simulink model "PID"  (R2023a)
settings: Solver=VariableStepAuto  StartTime=0  StopTime=5  RelTol=1e-3
model workspace (MAT data in the model file):
  mu = [0 0.4 0.8 0.97 1 0.98 0.96 0.94 0.92 0.9 0.88 0.855 0.83 0.81 0.79 0.77 0.75 0.73 0.72 0.71 0.7]
  slip = [0 0.05 0.1 0.15 0.2 0.25 0.3 0.35 0.4 0.45 0.5 0.55 0.6 0.65 0.7 0.75 0.8 0.85 0.9 0.95 1]
libraries: slpidlib x1, spsCurrentMeasurementLib x1, spsDCVoltageSourceLib x1, spsPermanentMagnetSynchronousMachineLib x1, spsUniversalBridgeLib x1, simulink x1, spspowerguiLib x1
settings Model: Creator=13524  LastModifiedBy=13524

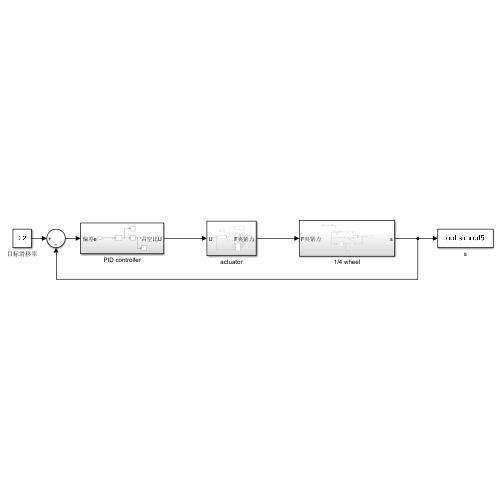
[thumbnail: Simulink's stored preview of the top-level diagram]
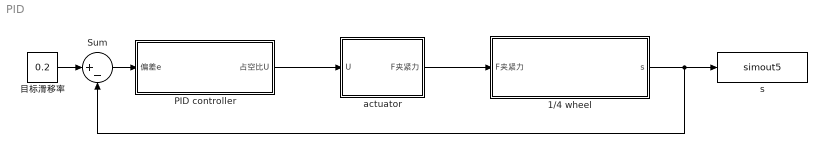
== system PID ==
  1/4 wheel : Subsystem
  PID controller : Subsystem
  Sum : Sum  Inputs=|+-
  actuator : Subsystem
  s : ToWorkspace  VariableName=simout5  SaveFormat=Timeseries  SampleTime=-1
  目标滑移率 : Constant  Value=0.2
  wires:
  1/4 wheel/1(s) -> s/1, Sum/2
  目标滑移率/1 -> Sum/1
  Sum/1 -> PID controller/1(偏差e)
  PID controller/1(占空比U) -> actuator/1(U)
  actuator/1(F夹紧力) -> 1/4 wheel/1(F夹紧力)

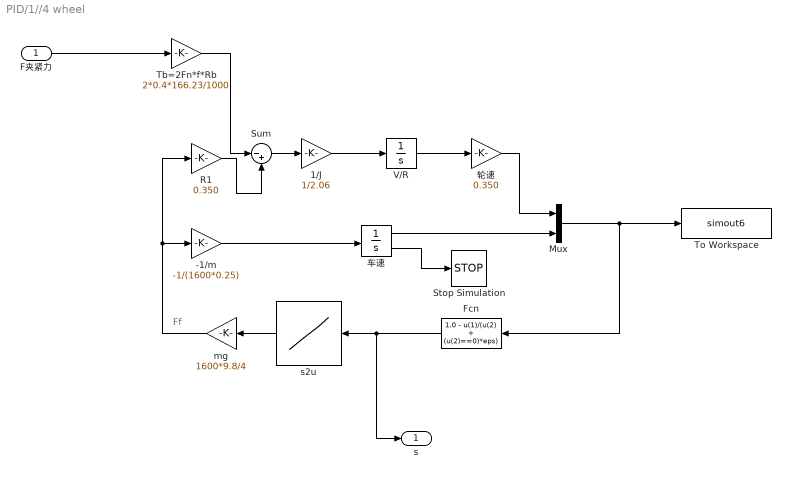
== system PID/1//4 wheel ==
  note: Ff
  F夹紧力 : Inport
  -1/m : Gain  Gain=-1/(1600*0.25)
  1/J : Gain  Gain=1/2.06
  Fcn : Fcn  Expr=1.0 - u(1)/(u(2) + (u(2)==0)*eps)
  Mux : Mux  Inputs=2
  R1 : Gain  Gain=0.350
  Stop Simulation : Stop
  Sum : Sum  Inputs=|-+
  Tb=2Fn*f*Rb : Gain  Gain=2*0.4*166.23/1000
  To Workspace : ToWorkspace  VariableName=simout6  SaveFormat=Timeseries  SampleTime=-1
  V/R : Integrator  InitialCondition=40/0.350  LimitOutput=on  UpperSaturationLimit=1000  LowerSaturationLimit=0
  mg : Gain  Gain=1600*9.8/4
  s2u : Lookup_n-D  NumberOfTableDimensions=1  BreakpointsForDimension1=[0;0.05;0.1;0.15;0.2;0.25;0.3;0.35;0.4;0.45;0.5;0.55;0.6;0.65;0.7;0.75;0.8;0.85;0.9;0.95;1]  Table=[0;0.4;0.8;0.97;1;0.98;0.96;0.94;0.92;0.9;0.88;0.855;0.83;0.81;0.79;0.77;0.75;0.73;0.72;0.71;0.7]  InternalRulePriority=Speed  RndMeth=Simplest
  车速 : Integrator  InitialCondition=40  LimitOutput=on  UpperSaturationLimit=100  LowerSaturationLimit=0  ShowSaturationPort=on
  轮速 : Gain  Gain=0.350
  s : Outport
  wires:
  V/R/1 -> 轮速/1
  轮速/1 -> Mux/1
  车速/1 -> Mux/2
  Mux/1 -> To Workspace/1, Fcn/1
  Fcn/1 -> s/1, s2u/1
  s2u/1 -> mg/1
  -1/m/1 -> 车速/1
  mg/1 -> R1/1, -1/m/1
  R1/1 -> Sum/2
  Sum/1 -> 1/J/1
  车速/2 -> Stop Simulation/1
  1/J/1 -> V/R/1
  F夹紧力/1 -> Tb=2Fn*f*Rb/1
  Tb=2Fn*f*Rb/1 -> Sum/1

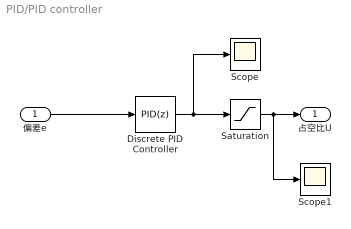
== system PID/PID controller ==
  偏差e : Inport
  Discrete PID Controller : slpidlib/PID Controller  Controller=PID  Form=Parallel  TimeDomain=Discrete-time  UseExternalTs=off  SampleTime=-1  IntegratorMethod=Forward Euler  FilterMethod=Forward Euler  ControllerParametersSource=internal  P=100  I=150  UseKiTs=off  D=0.2  N=100  UseFilter=off  TunerSelectOption=Transfer Function Based (PID Tuner App)  InitialConditionSource=internal  InitialConditionForIntegrator=0  InitialConditionForFilter=0  DifferentiatorICPrevScaledInput=0  ExternalReset=none  TrackingMode=off  Kt=1  LimitOutput=off  SatLimitsSource=internal  UpperSaturationLimit=inf  LowerSaturationLimit=-inf  LinearizeAsGain=off  AntiWindupMode=none  Kb=1  LimitIntegrator=off  UpperIntegratorSaturationLimit=inf  LowerIntegratorSaturationLimit=-inf  POutMin=[]  POutMax=[]  IOutMin=[]  IOutMax=[]  DOutMin=[]  DOutMax=[]  NOutMin=[]  NOutMax=[]  SumOutMin=[]  SumOutMax=[]  SaturationOutMin=[]  SaturationOutMax=[]  PParamMin=[]  PParamMax=[]  IParamMin=[]  IParamMax=[]  DParamMin=[]  DParamMax=[]  NParamMin=[]  NParamMax=[]  KbParamMin=[]  KbParamMax=[]  KtParamMin=[]  KtParamMax=[]  KbOutMin=[]  KbOutMax=[]  KtOutMin=[]  KtOutMax=[]  IntegratorOutMin=[]  IntegratorOutMax=[]  FilterOutMin=[]  FilterOutMax=[]  SumI1OutMin=[]  SumI1OutMax=[]  SumI2OutMin=[]  SumI2OutMax=[]  SumI3OutMin=[]  SumI3OutMax=[]  SumI4OutMin=[]  SumI4OutMax=[]  SumDOutMin=[]  SumDOutMax=[]  DifferentiatorOutMin=[]  DifferentiatorOutMax=[]  FilterDiffOutCoefMin=[]  FilterDiffOutCoefMax=[]  ReciprocalOutMin=[]  ReciprocalOutMax=[]  SumDenOutMin=[]  SumDenOutMax=[]  SumNumOutMin=[]  SumNumOutMax=[]  DivideOutMin=[]  DivideOutMax=[]  UdiffTsProdOutMin=[]  UdiffTsProdOutMax=[]  NTsProdOutMin=[]  NTsProdOutMax=[]  UintegralTsProdOutMin=[]  UintegralTsProdOutMax=[]  UngainTsProdOutMin=[]  UngainTsProdOutMax=[]  ClampingZeroOutDataTypeStr=Inherit: Inherit via back propagation  ClampingZeroOutMin=[]  ClampingZeroOutMax=[]  FilterDenConstantOutDataTypeStr=Inherit: Inherit via back propagation  FilterDenConstantOutMin=[]  FilterDenConstantOutMax=[]  PCopyOutDataTypeStr=Inherit: Inherit via back propagation  PCopyOutMin=[]  PCopyOutMax=[]  NCopyOutDataTypeStr=Inherit: Inherit via back propagation  NCopyOutMin=[]  NCopyOutMax=[]  IntegratorContinuousStateAttributes=''  IntegratorStateMustResolveToSignalObject=off  IntegratorRTWStateStorageClass=Auto  FilterContinuousStateAttributes=''  FilterStateMustResolveToSignalObject=off  FilterRTWStateStorageClass=Auto  ParallelPVariant=InternalParameters  IdealPVariant=Disabled  IVariant=InternalParameters  DVariant=InternalParameters  IntegratorVariant=Discrete  SatVariant=Disabled  AWVariant=Passthrough  PCopyVariant=Disabled  TRVariant=Disabled  FdbkBlocksVariant=Forward  IdealPFdbkVariant=Disabled  SatFdbkVariant=Disabled  DerivativeFilterVariant=Differentiator  NVariant=Passthrough  NCopyVariant=Disabled_SignalSpec  FilterICVariant=InternalICsDifferentiator  IntegratorICVariant=InternalICs  ExternalResetVariant=Disabled  TRSumVariant=Passthrough  SumFdbkVariant=Disabled  SumVariant=Sum_PID  TsampFilterVariant=InternalTs  TsampNgainVariant=Passthrough  TsampIntegralVariant=Disabled_SignalSpec  ExternalSaturationOutDataTypeStr=Inherit: Same as second input
      settings: LibrarySourceBlock=simulink/Discrete/Discrete PID Controller
  Saturation : Saturate  UpperLimit=4  LowerLimit=-4
  Scope : Scope
  Scope1 : Scope
  占空比U : Outport
  wires:
  偏差e/1 -> Discrete PID Controller/1
  Discrete PID Controller/1 -> Scope/1, Saturation/1
  Saturation/1 -> Scope1/1, 占空比U/1

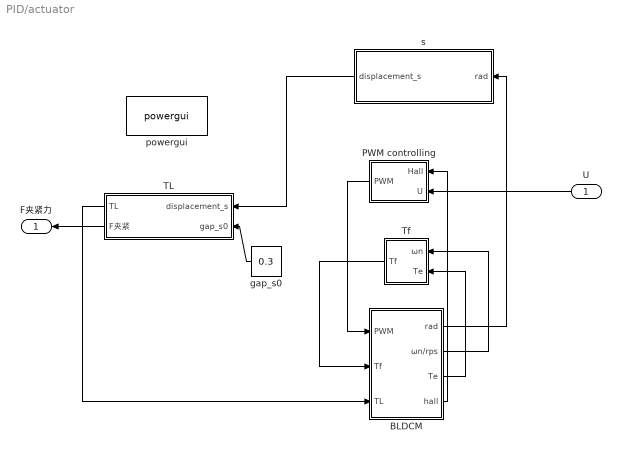
== system PID/actuator ==
  U : Inport
  BLDCM : Subsystem
  PWM controlling : Subsystem
  TL : Subsystem
  Tf : Subsystem
  gap_s0 : Constant  Value=0.3  VectorParams1D=off
  powergui : spspowerguiLib/powergui  Priority=1  SimulationMode=Discrete  SampleTime=0.0001  frequency=60  Iterations=50  frequencyindice=0  Pbase=100e6  ErrMax=1e-4  UnitsV=kV  UnitsW=MW  buscounter=0  FunctionMessages=off  echomessages=off  EnableUseOfTLC=off  CurrentSourceSwitches=off  DisableSnubberDevices=off  DisableRonSwitches=off  DisableVfSwitches=off  DisplayEquations=off  AutomaticDiscreteSolvers=off  SolverType=Tustin/Backward Euler (TBE)  Interpol=off  ExternalGateDelay=off  methode=off  Ts=100  x0status=blocks  SPID=on  SwTol=0  HookPort=off  NonlinearTolerance=1e-4  nMaxIteration=100  ContinueOnMaxIteration=off  RestoreLinks=warning  ResistiveCurrentMeasurement=off  Frange=[0:2:500]  Ylog=off  Xlog=on  ShowGrid=off  save=off  variable=ZData  structure=0  ZoomFFT=off  StartTime=0.0  cycles=1  DisplayStyle=1  fundamental=60  FreqAxis=off  MaxFrequency=1000  frequencyindicesteady=1  RmsSteady=1  display=off
  s : Subsystem
  F夹紧力 : Outport
  wires:
  PWM controlling/1(PWM) -> BLDCM/1(PWM)
  s/1(displacement_s) -> TL/1(displacement_s)
  BLDCM/4(hall) -> PWM controlling/1(Hall)
  Tf/1(Tf) -> BLDCM/2(Tf)
  TL/1(TL) -> BLDCM/3(TL)
  gap_s0/1 -> TL/2(gap_s0)
  BLDCM/1(rad) -> s/1(rad)
  BLDCM/3(Te) -> Tf/2(Te)
  BLDCM/2(ωn/rps) -> Tf/1(ωn)
  U/1 -> PWM controlling/2(U)
  TL/2(F夹紧) -> F夹紧力/1

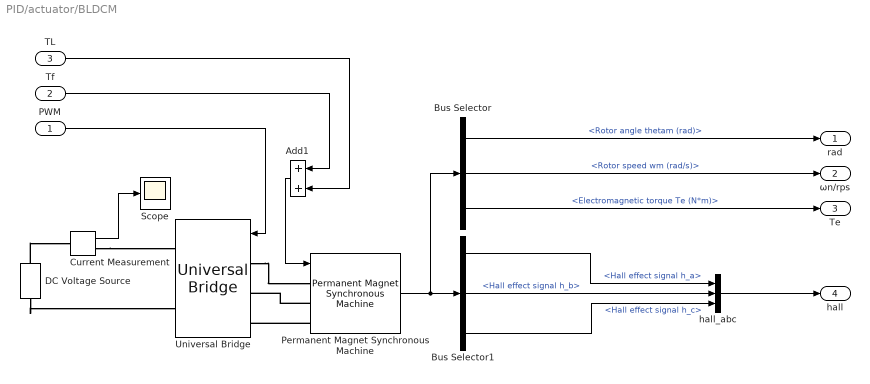
== system PID/actuator/BLDCM ==
  PWM : Inport
  Tf : Inport  Port=2
  TL : Inport  Port=3
  Add1 : Sum
  Bus Selector : BusSelector  OutputSignals=Rotor angle thetam (rad),Rotor speed wm (rad/s),Electromagnetic torque Te (N*m)
  Bus Selector1 : BusSelector  OutputSignals=Hall effect signal h_a,Hall effect signal h_b,Hall effect signal h_c
  Current Measurement : spsCurrentMeasurementLib/Current Measurement  PhasorSimulation=off  OutputType=Complex  PSBequivalent=0
  DC Voltage Source : spsDCVoltageSourceLib/DC Voltage Source  Amplitude=48  Measurements=Voltage
  Permanent Magnet Synchronous Machine : spsPermanentMagnetSynchronousMachineLib/Permanent Magnet Synchronous Machine  NbPhases=3  FluxDistribution=Trapezoidal  RotorType=Round  MechanicalLoad=Torque Tm  PresetModel=No  ShowDetailedParameters=on  MeasurementBus=off  Resistance=6.6  Inductance=0.99  dqInductances=[8.5e-3,8.5e-3]  La=0.000395  MachineConstant=Torque Constant (N.m / A_peak)  Flux=0.1405  VoltageCst=88.2788  TorqueCst=0.843  Flat=120  Mechanical=[0.00235 0.001086 3]  PolePairs=4  InitialConditions=[0,0,0,0]  InitialConditions5ph=[0 0 0 0 0 0]  RefAngle=Aligned with phase A axis (original Park)  IterativeDiscreteModel=Trapezoidal non iterative  TsBlock=-1  TsPowergui=0
  Scope : Scope
  Universal Bridge : spsUniversalBridgeLib/Universal Bridge  Arms=3  SnubberResistance=1e5  SnubberCapacitance=inf  Device=MOSFET / Diodes  Ron=1e-3  Lon=0  ForwardVoltages="[  0  0  ]"  ForwardVoltage=0  GTOparameters=[ 10e-6 , 20e-6 ]  IGBTparameters=[ 1e-6 , 2e-6 ]  Measurements=Device voltages  Measurements_2=None  converterType=Rectifier
  hall_abc : BusCreator  Inputs=3
  rad : Outport
  ωn/rps : Outport  Port=2
  Te : Outport  Port=3
  hall : Outport  Port=4
  wires:
  TL/1 -> Add1/2
  Bus Selector1/2 -> hall_abc/2  "<Hall effect signal h_b>"
  Add1/1 -> Permanent Magnet Synchronous Machine/1
  Bus Selector/3 -> Te/1  "<Electromagnetic torque Te (N*m)>"
  Bus Selector1/1 -> hall_abc/1  "<Hall effect signal h_a>"
  Permanent Magnet Synchronous Machine/1 -> Bus Selector/1, Bus Selector1/1
  Bus Selector1/3 -> hall_abc/3  "<Hall effect signal h_c>"
  Tf/1 -> Add1/1
  PWM/1 -> Universal Bridge/1
  Bus Selector/1 -> rad/1  "<Rotor angle thetam (rad)>"
  Bus Selector/2 -> ωn/rps/1  "<Rotor speed wm (rad/s)>"
  hall_abc/1 -> hall/1
  Current Measurement/1 -> Scope/1
  connections:
  Permanent Magnet Synchronous Machine/LConn3 -- Universal Bridge/LConn3
  Permanent Magnet Synchronous Machine/LConn2 -- Universal Bridge/LConn2
  Universal Bridge/LConn1 -- Permanent Magnet Synchronous Machine/LConn1
  DC Voltage Source/LConn1 -- Universal Bridge/RConn2
  DC Voltage Source/RConn1 -- Current Measurement/LConn1
  Current Measurement/RConn1 -- Universal Bridge/RConn1

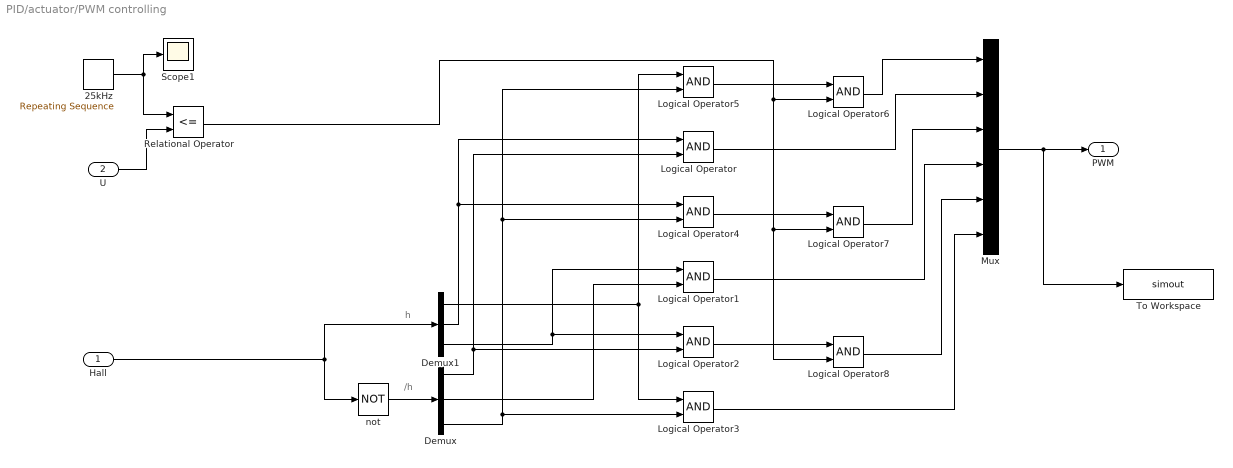
== system PID/actuator/PWM controlling ==
  note: h
  note: /h
  Hall : Inport
  U : Inport  Port=2
  25kHz : simulink/Sources/Repeating Sequence  rep_seq_t=[0 1/50000 1/25000]  rep_seq_y=[-4 4 -4]
  Demux : Demux  Outputs=3
  Demux1 : Demux  Outputs=3
  Logical Operator{,1..8} (9 alike) : Logic  AllPortsSameDT=off  OutDataTypeStr=boolean
  Mux : Mux  Inputs=6
  Relational Operator : RelationalOperator  Operator=<=  OutDataTypeStr=boolean  RndMeth=Simplest  InputSameDT=off
  Scope1 : Scope
  To Workspace : ToWorkspace  VariableName=simout  SaveFormat=Structure With Time  SampleTime=-1
  not : Logic  Operator=NOT  IconShape=distinctive  AllPortsSameDT=off  OutDataTypeStr=boolean
  PWM : Outport
  wires:
  Hall/1 -> not/1, Demux1/1
  Demux1/2 -> Logical Operator/1, Logical Operator4/1
  Demux/3 -> Logical Operator5/2, Logical Operator4/2, Logical Operator3/2
  Demux/1 -> Logical Operator/2, Logical Operator2/2
  Demux/2 -> Logical Operator1/2
  Logical Operator3/1 -> Mux/6
  Logical Operator7/1 -> Mux/3
  Relational Operator/1 -> Logical Operator6/2, Logical Operator7/2, Logical Operator8/2
  Demux1/1 -> Logical Operator5/1, Logical Operator3/1
  Demux1/3 -> Logical Operator1/1, Logical Operator2/1
  Logical Operator5/1 -> Logical Operator6/1
  Logical Operator8/1 -> Mux/5
  Logical Operator6/1 -> Mux/1
  Logical Operator2/1 -> Logical Operator8/1
  Logical Operator/1 -> Mux/2
  Logical Operator4/1 -> Logical Operator7/1
  Logical Operator1/1 -> Mux/4
  not/1 -> Demux/1
  U/1 -> Relational Operator/2
  25kHz/1 -> Scope1/1, Relational Operator/1
  Mux/1 -> To Workspace/1, PWM/1

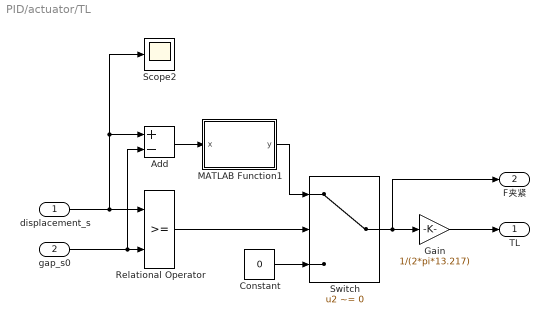
== system PID/actuator/TL ==
  displacement_s : Inport
  gap_s0 : Inport  Port=2
  Add : Sum  Inputs=+-
  Constant : Constant  Value=0
  Gain : Gain  Gain=1/(2*pi*13.217)
  MATLAB Function1 : MATLAB Function  TreatAsAtomicUnit=on
  Relational Operator : RelationalOperator  OutDataTypeStr=boolean  RndMeth=Simplest  InputSameDT=off
  Scope2 : Scope
  Switch : Switch  Criteria=u2 ~= 0  ZeroCross=off  SaturateOnIntegerOverflow=off  InputSameDT=off
  TL : Outport
  F夹紧 : Outport  Port=2
  wires:
  displacement_s/1 -> Scope2/1, Add/1, Relational Operator/1
  gap_s0/1 -> Add/2, Relational Operator/2
  Switch/1 -> F夹紧/1, Gain/1
  Constant/1 -> Switch/3
  Add/1 -> MATLAB Function1/1(x)
  MATLAB Function1/1(y) -> Switch/1
  Gain/1 -> TL/1
  Relational Operator/1 -> Switch/2

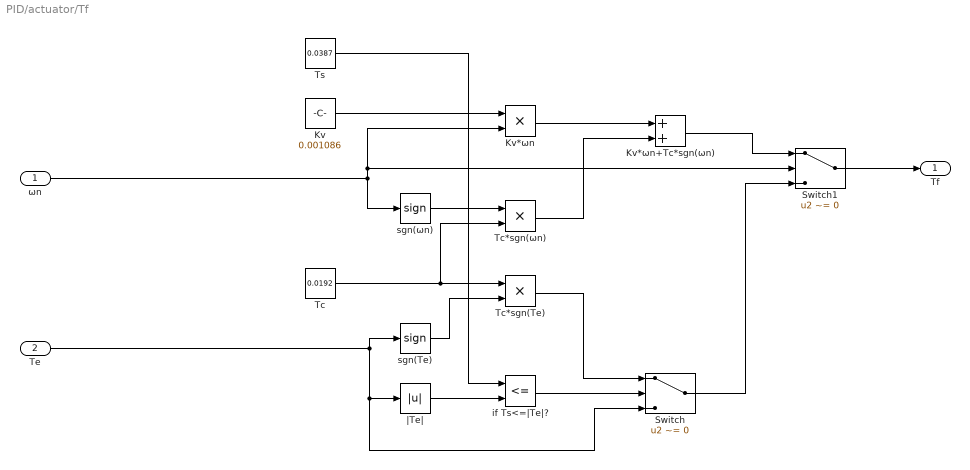
== system PID/actuator/Tf ==
  ωn : Inport
  Te : Inport  Port=2
  Kv : Constant  Value=0.001086
  Kv*ωn : Product
  Kv*ωn+Tc*sgn(ωn) : Sum
  Switch : Switch  Criteria=u2 ~= 0  SaturateOnIntegerOverflow=off  InputSameDT=off
  Switch1 : Switch  Criteria=u2 ~= 0  SaturateOnIntegerOverflow=off  InputSameDT=off
  Tc : Constant  Value=0.0192
  Tc*sgn(Te) : Product
  Tc*sgn(ωn) : Product
  Ts : Constant  Value=0.0387
  if Ts<=|Te|? : RelationalOperator  Operator=<=  OutDataTypeStr=boolean  RndMeth=Simplest  InputSameDT=off
  sgn(Te) : Signum
  sgn(ωn) : Signum
  |Te| : Abs  SaturateOnIntegerOverflow=off
  Tf : Outport
  wires:
  if Ts<=|Te|?/1 -> Switch/2
  Tc/1 -> Tc*sgn(ωn)/2, Tc*sgn(Te)/1
  Ts/1 -> if Ts<=|Te|?/1
  ωn/1 -> Switch1/2, Kv*ωn/2, sgn(ωn)/1
  Kv*ωn/1 -> Kv*ωn+Tc*sgn(ωn)/1
  Tc*sgn(ωn)/1 -> Kv*ωn+Tc*sgn(ωn)/2
  Kv*ωn+Tc*sgn(ωn)/1 -> Switch1/1
  |Te|/1 -> if Ts<=|Te|?/2
  Kv/1 -> Kv*ωn/1
  Tc*sgn(Te)/1 -> Switch/1
  sgn(ωn)/1 -> Tc*sgn(ωn)/1
  sgn(Te)/1 -> Tc*sgn(Te)/2
  Te/1 -> Switch/3, |Te|/1, sgn(Te)/1
  Switch/1 -> Switch1/3
  Switch1/1 -> Tf/1

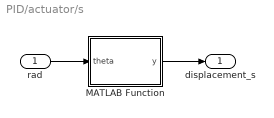
== system PID/actuator/s ==
  rad : Inport
  MATLAB Function : MATLAB Function  TreatAsAtomicUnit=on
  displacement_s : Outport
  wires:
  MATLAB Function/1(y) -> displacement_s/1
  rad/1 -> MATLAB Function/1(theta)

== matlab function PID/actuator/s/MATLAB Function ==
  data: theta input; y output
function y = fcn(theta)

y = theta/(2*pi*13.217);

== matlab function PID/actuator/TL/MATLAB Function1 ==
  data: x input; y output
function y = fcn(x)
y=-1805*x^3+27290*x^2-6036*x+376.2;
